simulink model "transformation_example"  (R2015a)
settings: Solver=ode45  StartTime=0.0  StopTime=0.08  RelTol=1e-3
InitFcn:
  | clear all;
  | close all;
libraries: powerlib_meascontrol x4, simulink_extras x2, simulink x1
settings Model: Creator=Dr Kashif  LastModifiedBy=Dr Kashif

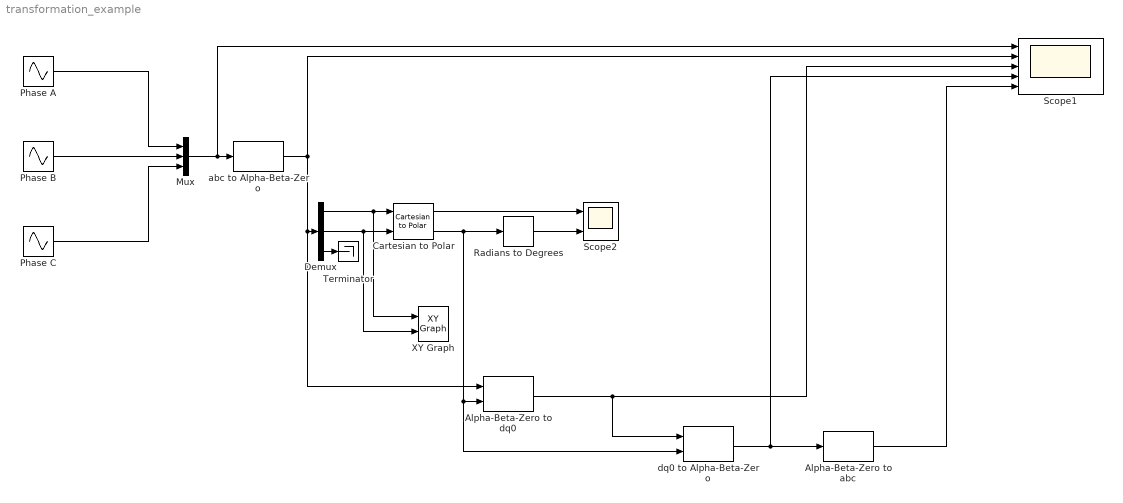
== system transformation_example ==
  Alpha-Beta-Zero to abc : powerlib_meascontrol/Transformations/Alpha-Beta-Zero to abc
  Alpha-Beta-Zero to dq0 : powerlib_meascontrol/Transformations/Alpha-Beta-Zero to dq0  Alignment=Aligned with phase A axis
  Cartesian to Polar : simulink_extras/Transformations/Cartesian to Polar
  Demux : Demux  Outputs=3
  Mux : Mux  Inputs=3
  Phase A : Sin  Frequency=50*2*pi  SampleTime=0
  Phase B : Sin  Frequency=50*2*pi  Phase=4*pi/3  SampleTime=0
  Phase C : Sin  Frequency=50*2*pi  Phase=2*pi/3  SampleTime=0
  Radians to Degrees : simulink_extras/Transformations/Radians to Degrees
  Scope1 : Scope  NumInputPorts=5
      settings: TimeRange=0.04  YMin=-1~-1.25~-0.25~-1.25~-1  YMax=1~1.25~1.25~1.25~1  SampleInput=on  SampleTime=10e-6
  Scope2 : Scope  NumInputPorts=2
      settings: TimeRange=0.04  YMin=0.95~-200  YMax=1.05~200  SampleInput=on  SampleTime=10e-6
  Terminator : Terminator
  XY Graph : simulink/Sinks/XY Graph  xmin=-1  xmax=1  ymin=-1  ymax=1  st=-1
  abc to Alpha-Beta-Zero : powerlib_meascontrol/Transformations/abc to Alpha-Beta-Zero
  dq0 to Alpha-Beta-Zero : powerlib_meascontrol/Transformations/dq0 to Alpha-Beta-Zero  Alignment=Aligned with phase A axis
  wires:
  Phase A/1 -> Mux/1
  Phase B/1 -> Mux/2
  Phase C/1 -> Mux/3
  abc to Alpha-Beta-Zero/1 -> Alpha-Beta-Zero to dq0/1, Demux/1, Scope1/2
  Mux/1 -> Scope1/1, abc to Alpha-Beta-Zero/1
  Demux/1 -> XY Graph/1, Cartesian to Polar/1
  Demux/2 -> XY Graph/2, Cartesian to Polar/2
  Cartesian to Polar/1 -> Scope2/1
  Cartesian to Polar/2 -> dq0 to Alpha-Beta-Zero/2, Alpha-Beta-Zero to dq0/2, Radians to Degrees/1
  Radians to Degrees/1 -> Scope2/2
  Alpha-Beta-Zero to dq0/1 -> dq0 to Alpha-Beta-Zero/1, Scope1/3
  Demux/3 -> Terminator/1
  dq0 to Alpha-Beta-Zero/1 -> Alpha-Beta-Zero to abc/1, Scope1/4
  Alpha-Beta-Zero to abc/1 -> Scope1/5
